simulink model "NGGenset_Test_System"  (Simulink 8.1)
settings: Solver=ode3  SolverMode=SingleTasking  StartTime=0.0  StopTime=150  FixedStep=Ts  RelTol=1e-3
model workspace (MAT data in the model file):
  op_snapshot1 : opcond.OperatingPoint (value not decoded)
PostLoadFcn:
  | Ts=50e-6;SIM_HIL=0;
InitFcn:
  | Ts=50e-6;SIM_HIL=0;
undefined symbols (not defined in the file or in its folder): Gen_900kW_external_control, HIL_GenSet, Left, type, V
libraries: powerlib x31, powerlib_extras x24, simulink x10, dspsigops x6, breakers_1ph_3ph x6, rtio_generic_modbus x6, cables_lib x5, rtlab x2, ssn_lib x2, artemis x1, NG_Genset_lib x1
(part 1 of 3)
settings Model: ARTEMISmethode_block_infos=$$__separator__$$NGGenset_Test_System/ARTEMIS Guide$$__separator__$$  Creator=CH24070  LastModifiedBy=ed12083
settings OptimizationCC: BlockReduction=off  BooleanDataType=off  ExpressionDepthLimit=128
settings DebuggingCC: SaveWithParameterizedLinksMsg=none  SignalResolutionControl=TryResolveAllWithWarning  SolverPrmCheckMsg=none  MultiTaskDSMMsg=warning  MultiTaskCondExecSysMsg=none  FcnCallInpInsideContextMsg=EnableAllAsError  StrictBusMsg=None
settings HardwareCC: TargetUnknown=on
settings RTWCC: IncludeERTFirstTime=on
settings GRTTargetCC: CombineOutputUpdateFcns=on  GRTInterface=off

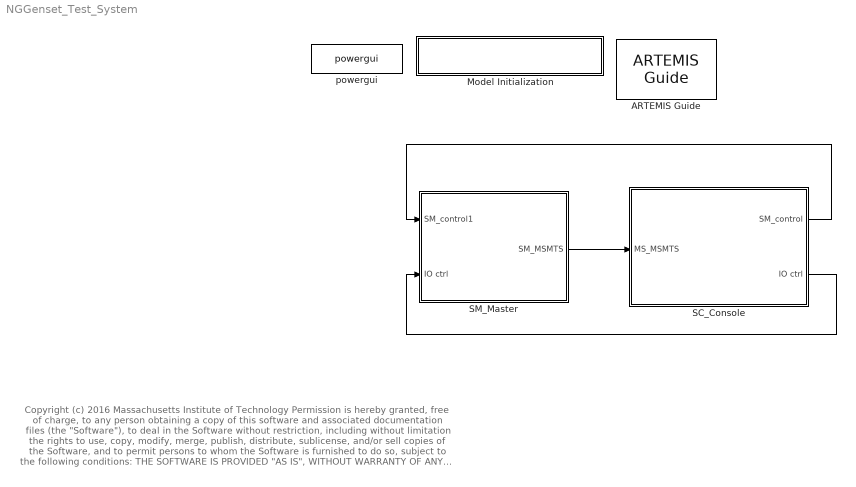
== system NGGenset_Test_System ==
  note: Copyright (c) 2016 Massachusetts Institute of Technology
      | Permission is hereby granted, free of charge, to any person obtaining a copy of this software and associated documentation files (the "Software"), to deal
      | in the Software without restriction, including without limitation the rights to use, copy, modify, merge, publish, distribute, sublicense, and/or sell copies of the
      | Software, and to permit persons to whom the Software is furnished to do so, subject to the following conditions:
      |
      | THE SOFTWARE IS PROVIDED "AS IS", WITHOUT WARRANTY OF ANY KIND, EXPRESS OR IMPLIED, INCLUDING BUT NOT LIMITED TO THE
      | WARRANTIES OF MERCHANTABILITY, FITNESS FOR A PARTICULAR PURPOSE AND NONINFRINGEMENT. IN NO EVENT SHALL THE AUTHORS
      | OR COPYRIGHT HOLDERS BE LIABLE FOR ANY CLAIM, DAMAGES OR OTHER LIABILITY, WHETHER IN AN ACTION OF CONTRACT, TORT OR
      | OTHERWISE, ARISING FROM, OUT OF OR IN CONNECTION WITH THE SOFTWARE OR THE USE OR OTHER DEALINGS IN THE SOFTWARE.
  ARTEMIS Guide : artemis/ARTEMIS/ARTEMIS Guide  Tag=FTSSmethode_opal_4hx0r99  Description=5.0_z1  lock=on  Ts=Ts  opt=art5  dyna=off  nb_perm=4  RT_fullcomp=off  ssn=on  ssn_itvc=off  ssn_ivic=off  ssn_ext=off  ssn_solver=Art5 with Backward Euler nodal interface  ssn_impulse=off  ssn_quasimpulse=off  ssn_impulse_loop=2  paraExtinctionThy=off  Thy_Impulse=on  dtc=Off  dtc_opt=normal  ao=on  simtype=off  ct_mac=off  lin_mov=off  lsp=[0.001 2]  spike_skip=Disabled  dtc_extra=1  dtc_sws=normal  dtc_pied=0.5  SPSRulesBlock=SPSRules  tre=on  ctmm=off  LF=off  dpl_type=ARTEMiS DPL  rlc_type=off  custom_type=off  para=on  ssn_ImpulseLoopBlockedStateUpdate=2  ssn_mov_iter_number=5  ssn_switch_iter_number=5
  Model Initialization : Subsystem  AncestorBlock=artemis/Tools /Misc/Model Initialization  mask(Model Functions){InitFcnX=Ts=50e-6;SIM_HIL=0;, prel=off, posl=on, inif=on, strf=off}
      mask prompts: InitFcnX "Initialisation"; prel "Preload Function"; posl "PostLoad Function"; inif "InitFcn"; strf "StartFcn"
      mask init:
      | currentBlock = gcb;
      | root = bdroot(currentBlock);
      | 
      | if ~strcmp(get_param(root,'BlockDiagramType'),'library')
      |     if prel==1
      |         set_param(root, 'PreLoadFcn', InitFcnX);
      |     else
      |         set_param(root, 'PreLoadFcn', '');
      |     end
      |     if inif==1
      |         set_param(root, 'InitFcn', InitFcnX);
      |     else
      |         set_param(root, 'InitFcn', '');
      |     end
      |     if strf==1
      |         set_param(root, 'StartFcn', InitFcnX);
      |     else
      |         set_param(root, 'StartFcn', '');
      |     end
      |     if posl==1
      |         set_param(root, 'PostLoadFcn', InitFcnX);
      |     else
      |         set_param(root, 'PostLoadFcn', '');
      |     end
      | end
      | 
      | pos = get_param(currentBlock, 'Position');
      | width = pos(3) - pos(1); height = pos(4) - pos(2);
      | txt = [ upper(root) '\n' '- InitFcn. . . . . '  get_param(root, 'InitFcn') ];
      settings: CopyFcn=set_param(gcb,'LinkStatus','inactive')
      mask Display: text(5, height*0.5, txt, 'horizontalAlignment', 'left', 'verticalAlignment', 'middle') ;
  SC_Console : Subsystem
  SM_Master : Subsystem
  powergui : powerlib/powergui  Priority=2  SimulationMode=Discrete  SolverType=Tustin  SampleTime=Ts  frequency=60  SPID=off  DisableSnubberDevices=off  DisableRonSwitches=off  DisableVfSwitches=off  SwTol=0  Interpol=off  DisplayEquations=off  frequencyindice=60  Pbase=100e6  ErrMax=1e-4  Iterations=50  UnitsV=kV  UnitsW=MW  FunctionMessages=off  echomessages=off  HookPort=off  EnableUseOfTLC=off  x0status=blocks  RestoreLinks=warning  ResistiveCurrentMeasurement=off  Frange=logspace(0,3,50)  Ylog=off  Xlog=off  ShowGrid=off  save=off  variable=ZData  structure=0  ZoomFFT=on  StartTime=0.0  cycles=2  DisplayStyle=off  fundamental=60  FreqAxis=off  MaxFrequency=1000  frequencyindicesteady=1  RmsSteady=1  display=off  Ts=0  methode=off
  wires:
  SM_Master/1(SM_MSMTS) -> SC_Console/1(MS_MSMTS)
  SC_Console/1(SM_control) -> SM_Master/1(SM_control1)
  SC_Console/2(IO ctrl) -> SM_Master/2(IO ctrl)

== system NGGenset_Test_System/Model Initialization ==

== system NGGenset_Test_System/SC_Console ==
  note: The 'Overruns' value should remain at 0.
      | The 'Ttotal' value should be equal to the
      | model Fixed-Step size.
  MS_MSMTS : Inport
  Bus Selector : BusSelector  OutputSignals=Grid_PRM,Mains1_PRM,GEN_3_5MVA_PRM,Gen1_meas,Digital In,Load1,Load2,Load3,signal12
  Bus Selector{1..4,7..8} (6 alike) : BusSelector  OutputSignals=Grid_Status,sel_787.Grid_Vabc,sel_787.Iabc,sel_787.Grid_P,sel_787.Grid_Q
  Gen1_3.5MVA : Subsystem  AncestorBlock=HIL_GenSet/Gen_900kW_external_control
  OpComm : rtlab/OpComm  nbport=1  groupe_acq=1  subsys_rate=0  st=0  Synchronization=on  Interpolation=on  Threshold=1.0  Missed_Data=off  Sim_Time=off  Samples=off  dynSigOut=off  from_console=0  warning_done=off  writeOpCommFile=off  Offset=off
  Scope Gen1 : Scope  NumInputPorts=4
      settings: ShowLegends=on  TimeRange=150  YMin=-12500~-1100~-1.5e+06~-1.1e+07  YMax=12500~900~600000~1e+06  Decimation=100
  Scope Grid : Scope  NumInputPorts=5
      settings: TimeRange=60  YMin=0~-20000~-20000~-1000000~-1000000  YMax=1~20000~20000~4000000~4000000  SaveName=ScopeData7  Decimation=100
  Scope Load1 : Scope  NumInputPorts=5
      settings: TimeRange=60  YMin=0~-600~-2000~-1000000~-1000000  YMax=1~600~2000~1000000~1000000  SaveName=ScopeData6  Decimation=100
  Scope Load2 : Scope  NumInputPorts=5
      settings: TimeRange=60  YMin=0~-600~-2000~-1000000~-1000000  YMax=1~600~2000~1000000~1000000  SaveName=ScopeData11  Decimation=100
  Scope Load3 : Scope  NumInputPorts=5
      settings: TimeRange=60  YMin=0~-600~-2000~-1000000~-1000000  YMax=1~600~2000~1000000~1000000  SaveName=ScopeData10  Decimation=100
  Scope Mains1 : Scope  NumInputPorts=5
      settings: TimeRange=60  YMin=0~-20000~-20000~-1000000~-1000000  YMax=1~20000~20000~4000000~4000000  SaveName=ScopeData5  Decimation=100
  Woodward : Subsystem
  SM_control : Outport
  IO ctrl : Outport  Port=2
  wires:
  MS_MSMTS/1 -> OpComm/1
  Gen1_3.5MVA/1(S) -> SM_control/1  "Gen1_3.5MVA"
  OpComm/1 -> Bus Selector/1
  Woodward/1(Out1) -> IO ctrl/1
  Bus Selector1/1 -> Scope Grid/1  "<Grid_Status>"
  Bus Selector1/2 -> Scope Grid/2  "<Grid_Vabc>"
  Bus Selector1/3 -> Scope Grid/3  "<Iabc>"
  Bus Selector1/4 -> Scope Grid/4  "<Grid_P>"
  Bus Selector1/5 -> Scope Grid/5  "<Grid_Q>"
  Bus Selector2/1 -> Scope Mains1/1  "<Grid_Status>"
  Bus Selector2/2 -> Scope Mains1/2  "<Grid_Vabc>"
  Bus Selector2/3 -> Scope Mains1/3  "<Iabc>"
  Bus Selector2/4 -> Scope Mains1/4  "<Grid_P>"
  Bus Selector2/5 -> Scope Mains1/5  "<Grid_Q>"
  Bus Selector/1 -> Bus Selector1/1  "<Grid_PRM>"
  Bus Selector/2 -> Bus Selector2/1  "<Mains1_PRM>"
  Bus Selector3/1 -> Scope Load1/1  "<Grid_Status>"
  Bus Selector3/2 -> Scope Load1/2  "<Grid_Vabc>"
  Bus Selector3/3 -> Scope Load1/3  "<Iabc>"
  Bus Selector3/4 -> Scope Load1/4  "<Grid_P>"
  Bus Selector3/5 -> Scope Load1/5  "<Grid_Q>"
  Bus Selector/6 -> Bus Selector3/1  "<Load1>"
  Bus Selector4/2 -> Scope Gen1/1  "<Grid_Vabc>"
  Bus Selector4/3 -> Scope Gen1/2  "<Iabc>"
  Bus Selector4/4 -> Scope Gen1/3  "<Grid_P>"
  Bus Selector4/5 -> Scope Gen1/4  "<Grid_Q>"
  Bus Selector/3 -> Bus Selector4/1  "<GEN_3_5MVA_PRM>"
  Bus Selector/4 -> Woodward/1(Gen1_Primary)  "<Gen1_meas>"
  Bus Selector/5 -> Woodward/2(DIn_Ch00_31)  "<Digital In>"
  Bus Selector7/1 -> Scope Load3/1  "<Grid_Status>"
  Bus Selector7/2 -> Scope Load3/2  "<Grid_Vabc>"
  Bus Selector7/3 -> Scope Load3/3  "<Iabc>"
  Bus Selector7/4 -> Scope Load3/4  "<Grid_P>"
  Bus Selector7/5 -> Scope Load3/5  "<Grid_Q>"
  Bus Selector8/1 -> Scope Load2/1  "<Grid_Status>"
  Bus Selector8/2 -> Scope Load2/2  "<Grid_Vabc>"
  Bus Selector8/3 -> Scope Load2/3  "<Iabc>"
  Bus Selector8/4 -> Scope Load2/4  "<Grid_P>"
  Bus Selector8/5 -> Scope Load2/5  "<Grid_Q>"
  Bus Selector/8 -> Bus Selector7/1  "<Load3>"
  Bus Selector/7 -> Bus Selector8/1  "<Load2>"

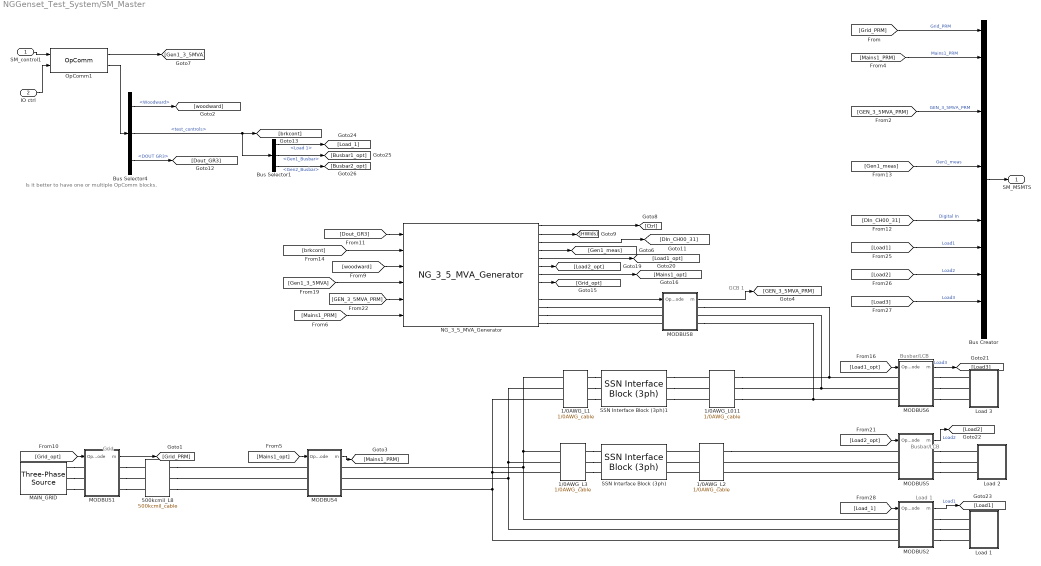
== system NGGenset_Test_System/SM_Master ==
  note: Is it better to have one
      | or multiple OpComm blocks.
  note: GCB 1
  note: Busbar/LCB
  note: Grid
  note: Load 1
  note: Busbar/LCB
  SM_control1 : Inport
  IO ctrl : Inport  Port=2
  1/0AWG_L011 : cables_lib/1//0AWG_cable  length=1000  par_sets=1
  1/0AWG_L1 : cables_lib/1//0AWG_cable  length=1  par_sets=1
  1/0AWG_L2 : cables_lib/1//0AWG_cable  length=1  par_sets=1
  1/0AWG_L3 : cables_lib/1//0AWG_cable  length=1  par_sets=1
  500kcmil_L8 : cables_lib/500kcmil_cable  length=1  par_sets=1
  Bus Creator : BusCreator  Inputs=12
  Bus Selector1 : BusSelector  OutputSignals=Load 1,Gen1_Busbar,Gen2_Busbar
  Bus Selector4 : BusSelector  OutputSignals=Woodward,test_controls,DOUT GR3
  Load 1 : Subsystem  mask{v=13800, kVA=3500*.5, pf=0.90}
      mask prompts: v "VRMSLL"
  Load 2 : Subsystem  mask{v=13800, kVA=3500*.4, pf=0.90}
      mask prompts: v "VRMSLL"
  Load 3 : Subsystem  mask{v=13800, kVA=3500*.1, pf=0.90}
      mask prompts: v "VRMSLL"
  MAIN_GRID : powerlib/Electrical Sources/Three-Phase Source  Voltage=13800  PhaseAngle=0  Frequency=60  InternalConnection=Yg  SpecifyImpedance=on  Resistance=0.8929  Inductance=16.58e-3  ShortCircuitLevel=375e6  BaseVoltage=13800  XRratio=7.9  BusType=swing  Pref=0  Qref=0  Qmin=-inf  Qmax=inf
  MODBUS1 : Subsystem  AncestorBlock=breakers_1ph_3ph/Protection  mask(Protection and Metering){IOC=15E3, TOC=1800, Ts=Ts, VRMSLL=13800, I_nom=200}
      mask prompts: IOC "IOC setting [A]"; TOC "TOC setting [A]"; Ts "Sampling Time [Sec]"; VRMSLL "Nominal Voltage [VRMSLL]"; I_nom "Continous Current [A]"
      mask help:
      | This block simulates the behavior of selected relay functions as well as metering equipment.
      | The block is intended to communicate with a microgrid controller providing it measurements, and switching controls.
      |
      | Supported relay functions (as of 06-15-2015):
      | 50/51: instantaneous and time-inverse overcurrent protection (moderate curve)
      mask Help:
      | This block simulates the behavior of selected relay functions as well as metering equipment (60 Hz - only).
      | The block is intended to communicate with a microgrid controller providing it measurements, and switching controls.
      | 
      | Supported relay functions (as of 06-15-2015):
      | 50/51: instantaneous and time-inverse overcurrent protection (moderate curve)
      | 
      | The input parameters are:
      | 0) Ts:  Sampling time [Seconds]
      | 1) State: 0 for relay logic mode, 1 to close the controlled breaker/switch,
      | and 2 to open the controlled breaker/switch
      | 2) TOC: Time-inverse overcurrent setting [Amperes]
      | 3) IOC: Instantaneous overcurrent setting [Amperes]
      | 
      | Metered parameters are:
      | 0) Status (0-closed, 1-open)
      | 1) Instantaneous voltage (abc)
      | 2) Instantaneous current (abc)
  MODBUS2 : Subsystem  AncestorBlock=breakers_1ph_3ph/Protection  mask(Protection and Metering){IOC=15E3, TOC=1800, Ts=Ts, VRMSLL=13800, I_nom=200}
      mask prompts: IOC "IOC setting [A]"; TOC "TOC setting [A]"; Ts "Sampling Time [Sec]"; VRMSLL "Nominal Voltage [VRMSLL]"; I_nom "Continous Current [A]"
      mask help:
      | This block simulates the behavior of selected relay functions as well as metering equipment.
      | The block is intended to communicate with a microgrid controller providing it measurements, and switching controls.
      |
      | Supported relay functions (as of 06-15-2015):
      | 50/51: instantaneous and time-inverse overcurrent protection (moderate curve)
      mask Help:
      | This block simulates the behavior of selected relay functions as well as metering equipment (60 Hz - only).
      | The block is intended to communicate with a microgrid controller providing it measurements, and switching controls.
      | 
      | Supported relay functions (as of 06-15-2015):
      | 50/51: instantaneous and time-inverse overcurrent protection (moderate curve)
      | 
      | The input parameters are:
      | 0) Ts:  Sampling time [Seconds]
      | 1) State: 0 for relay logic mode, 1 to close the controlled breaker/switch,
      | and 2 to open the controlled breaker/switch
      | 2) TOC: Time-inverse overcurrent setting [Amperes]
      | 3) IOC: Instantaneous overcurrent setting [Amperes]
      | 
      | Metered parameters are:
      | 0) Status (0-closed, 1-open)
      | 1) Instantaneous voltage (abc)
      | 2) Instantaneous current (abc)
  MODBUS4 : Subsystem  AncestorBlock=breakers_1ph_3ph/Protection  mask(Protection and Metering){IOC=15E3, TOC=1800, Ts=Ts, VRMSLL=13800, I_nom=2000}
      mask prompts: IOC "IOC setting [A]"; TOC "TOC setting [A]"; Ts "Sampling Time [Sec]"; VRMSLL "Nominal Voltage [VRMSLL]"; I_nom "Continous Current [A]"
      mask help:
      | This block simulates the behavior of selected relay functions as well as metering equipment.
      | The block is intended to communicate with a microgrid controller providing it measurements, and switching controls.
      |
      | Supported relay functions (as of 06-15-2015):
      | 50/51: instantaneous and time-inverse overcurrent protection (moderate curve)
      mask Help:
      | This block simulates the behavior of selected relay functions as well as metering equipment (60 Hz - only).
      | The block is intended to communicate with a microgrid controller providing it measurements, and switching controls.
      | 
      | Supported relay functions (as of 06-15-2015):
      | 50/51: instantaneous and time-inverse overcurrent protection (moderate curve)
      | 
      | The input parameters are:
      | 0) Ts:  Sampling time [Seconds]
      | 1) State: 0 for relay logic mode, 1 to close the controlled breaker/switch,
      | and 2 to open the controlled breaker/switch
      | 2) TOC: Time-inverse overcurrent setting [Amperes]
      | 3) IOC: Instantaneous overcurrent setting [Amperes]
      | 
      | Metered parameters are:
      | 0) Status (0-closed, 1-open)
      | 1) Instantaneous voltage (abc)
      | 2) Instantaneous current (abc)
  MODBUS5 : Subsystem  AncestorBlock=breakers_1ph_3ph/Protection  mask(Protection and Metering){IOC=15E3, TOC=1800, Ts=Ts, VRMSLL=13800, I_nom=200}
      mask prompts: IOC "IOC setting [A]"; TOC "TOC setting [A]"; Ts "Sampling Time [Sec]"; VRMSLL "Nominal Voltage [VRMSLL]"; I_nom "Continous Current [A]"
      mask help:
      | This block simulates the behavior of selected relay functions as well as metering equipment.
      | The block is intended to communicate with a microgrid controller providing it measurements, and switching controls.
      |
      | Supported relay functions (as of 06-15-2015):
      | 50/51: instantaneous and time-inverse overcurrent protection (moderate curve)
      mask Help:
      | This block simulates the behavior of selected relay functions as well as metering equipment (60 Hz - only).
      | The block is intended to communicate with a microgrid controller providing it measurements, and switching controls.
      | 
      | Supported relay functions (as of 06-15-2015):
      | 50/51: instantaneous and time-inverse overcurrent protection (moderate curve)
      | 
      | The input parameters are:
      | 0) Ts:  Sampling time [Seconds]
      | 1) State: 0 for relay logic mode, 1 to close the controlled breaker/switch,
      | and 2 to open the controlled breaker/switch
      | 2) TOC: Time-inverse overcurrent setting [Amperes]
      | 3) IOC: Instantaneous overcurrent setting [Amperes]
      | 
      | Metered parameters are:
      | 0) Status (0-closed, 1-open)
      | 1) Instantaneous voltage (abc)
      | 2) Instantaneous current (abc)
  MODBUS6 : Subsystem  AncestorBlock=breakers_1ph_3ph/Protection  mask(Protection and Metering){IOC=15E3, TOC=1800, Ts=Ts, VRMSLL=13800, I_nom=200}
      mask prompts: IOC "IOC setting [A]"; TOC "TOC setting [A]"; Ts "Sampling Time [Sec]"; VRMSLL "Nominal Voltage [VRMSLL]"; I_nom "Continous Current [A]"
      mask help:
      | This block simulates the behavior of selected relay functions as well as metering equipment.
      | The block is intended to communicate with a microgrid controller providing it measurements, and switching controls.
      |
      | Supported relay functions (as of 06-15-2015):
      | 50/51: instantaneous and time-inverse overcurrent protection (moderate curve)
      mask Help:
      | This block simulates the behavior of selected relay functions as well as metering equipment (60 Hz - only).
      | The block is intended to communicate with a microgrid controller providing it measurements, and switching controls.
      | 
      | Supported relay functions (as of 06-15-2015):
      | 50/51: instantaneous and time-inverse overcurrent protection (moderate curve)
      | 
      | The input parameters are:
      | 0) Ts:  Sampling time [Seconds]
      | 1) State: 0 for relay logic mode, 1 to close the controlled breaker/switch,
      | and 2 to open the controlled breaker/switch
      | 2) TOC: Time-inverse overcurrent setting [Amperes]
      | 3) IOC: Instantaneous overcurrent setting [Amperes]
      | 
      | Metered parameters are:
      | 0) Status (0-closed, 1-open)
      | 1) Instantaneous voltage (abc)
      | 2) Instantaneous current (abc)
  MODBUS8 : Subsystem  AncestorBlock=breakers_1ph_3ph/Protection  mask(Protection and Metering){IOC=15E3, TOC=1800, Ts=Ts, VRMSLL=13800, I_nom=2000}
      mask prompts: IOC "IOC setting [A]"; TOC "TOC setting [A]"; Ts "Sampling Time [Sec]"; VRMSLL "Nominal Voltage [VRMSLL]"; I_nom "Continous Current [A]"
      mask help:
      | This block simulates the behavior of selected relay functions as well as metering equipment.
      | The block is intended to communicate with a microgrid controller providing it measurements, and switching controls.
      |
      | Supported relay functions (as of 06-15-2015):
      | 50/51: instantaneous and time-inverse overcurrent protection (moderate curve)
      mask Help:
      | This block simulates the behavior of selected relay functions as well as metering equipment (60 Hz - only).
      | The block is intended to communicate with a microgrid controller providing it measurements, and switching controls.
      | 
      | Supported relay functions (as of 06-15-2015):
      | 50/51: instantaneous and time-inverse overcurrent protection (moderate curve)
      | 
      | The input parameters are:
      | 0) Ts:  Sampling time [Seconds]
      | 1) State: 0 for relay logic mode, 1 to close the controlled breaker/switch,
      | and 2 to open the controlled breaker/switch
      | 2) TOC: Time-inverse overcurrent setting [Amperes]
      | 3) IOC: Instantaneous overcurrent setting [Amperes]
      | 
      | Metered parameters are:
      | 0) Status (0-closed, 1-open)
      | 1) Instantaneous voltage (abc)
      | 2) Instantaneous current (abc)
  NG_3_5_MVA_Generator : NG_Genset_lib/NG_3_5_MVA_Generator
  OpComm1 : rtlab/OpComm  nbport=2  groupe_acq=1  subsys_rate=0  st=0  Synchronization=on  Interpolation=on  Threshold=1.0  Missed_Data=off  Sim_Time=off  Samples=off  dynSigOut=off  from_console=1  warning_done=off  writeOpCommFile=off  Offset=off
  SSN Interface Block (3ph) : ssn_lib/SSN Interface Block (3ph)  nb_phase=3  nb_port=2  p1_type=V-type(Left)  p2_type=V-type (Right)  p3_type=V-type(Left)  p4_type=V-type(Left)  p5_type=V-type(Left)  p6_type=V-type(Left)  p7_type=V-type(Left)  p8_type=V-type(Left)  p9_type=V-type(Left)  p10_type=V-type(Left)  p11_type=V-type(Left)  p12_type=V-type(Left)  p13_type=V-type(Left)  p14_type=V-type(Left)  p15_type=V-type(Left)  p16_type=V-type(Left)  I_port_shunt_resistance=1e9
  SSN Interface Block (3ph)1 : ssn_lib/SSN Interface Block (3ph)  nb_phase=3  nb_port=2  p1_type=V-type(Left)  p2_type=V-type (Right)  p3_type=V-type(Left)  p4_type=V-type(Left)  p5_type=V-type(Left)  p6_type=V-type(Left)  p7_type=V-type(Left)  p8_type=V-type(Left)  p9_type=V-type(Left)  p10_type=V-type(Left)  p11_type=V-type(Left)  p12_type=V-type(Left)  p13_type=V-type(Left)  p14_type=V-type(Left)  p15_type=V-type(Left)  p16_type=V-type(Left)  I_port_shunt_resistance=1e9
  SM_MSMTS : Outport
  wires:
  [Grid_PRM] -> Bus Creator/1  "Grid_PRM"
  [GEN_3_5MVA_PRM] -> Bus Creator/4  "GEN_3_5MVA_PRM"
  [Mains1_PRM] -> Bus Creator/2  "Mains1_PRM"
  Bus Creator/1 -> SM_MSMTS/1
  SM_control1/1 -> OpComm1/1
  OpComm1/1 -> [Gen1_3_5MVA]
  OpComm1/2 -> Bus Selector4/1
  Bus Selector4/1 -> [woodward]  "<Woodward>"
  IO ctrl/1 -> OpComm1/2
  Bus Selector4/3 -> [Dout_GR3]  "<DOUT GR3>"
  Bus Selector4/2 -> [brkcont], Bus Selector1/1  "<test_controls>"
  MODBUS1/1(m) -> [Grid_PRM]
  MODBUS8/1(m) -> [GEN_3_5MVA_PRM]
  [Dout_GR3] -> NG_3_5_MVA_Generator/1
  [brkcont] -> NG_3_5_MVA_Generator/2
  NG_3_5_MVA_Generator/4 -> [Gen1_meas]
  NG_3_5_MVA_Generator/1 -> [Ctrl]
  NG_3_5_MVA_Generator/2 -> [HWIds]
  NG_3_5_MVA_Generator/3 -> [DIn_CH00_31]
  [Gen1_3_5MVA] -> NG_3_5_MVA_Generator/4
  [woodward] -> NG_3_5_MVA_Generator/3
  NG_3_5_MVA_Generator/10 -> MODBUS8/1(Op_Mode)
  [Gen1_meas] -> Bus Creator/6  "Gen1_meas"
  [DIn_CH00_31] -> Bus Creator/8  "Digital In"
  NG_3_5_MVA_Generator/8 -> [Grid_opt]
  [Grid_opt] -> MODBUS1/1(Op_Mode)
  NG_3_5_MVA_Generator/7 -> [Mains1_opt]
  [Mains1_PRM] -> NG_3_5_MVA_Generator/6
  NG_3_5_MVA_Generator/6 -> [Load2_opt]
  NG_3_5_MVA_Generator/5 -> [Load1_opt]
  [GEN_3_5MVA_PRM] -> NG_3_5_MVA_Generator/5
  MODBUS4/1(m) -> [Mains1_PRM]
  [Mains1_opt] -> MODBUS4/1(Op_Mode)
  [Load2_opt] -> MODBUS5/1(Op_Mode)
  [Load1_opt] -> MODBUS6/1(Op_Mode)
  MODBUS2/1(m) -> [Load1]  "Load1"
  MODBUS5/1(m) -> [Load2]  "Load2"
  MODBUS6/1(m) -> [Load3]  "Load3"
  [Load1] -> Bus Creator/9  "Load1"
  [Load2] -> Bus Creator/10  "Load2"
  [Load3] -> Bus Creator/11  "Load3"
  Bus Selector1/1 -> [Load_1]  "<Load 1>"
  Bus Selector1/2 -> [Busbar1_opt]  "<Gen1_Busbar>"
  Bus Selector1/3 -> [Busbar2_opt]  "<Gen2_Busbar>"
  [Load_1] -> MODBUS2/1(Op_Mode)
  connections:
  500kcmil_L8/RConn1 -- MODBUS4/LConn1
  500kcmil_L8/RConn2 -- MODBUS4/LConn2
  500kcmil_L8/RConn3 -- MODBUS4/LConn3
  MODBUS8/RConn3 -- MODBUS6/LConn3 -- 1/0AWG_L011/RConn3
  MODBUS1/RConn3 -- 500kcmil_L8/LConn3
  MODBUS1/RConn2 -- 500kcmil_L8/LConn2
  MAIN_GRID/RConn3 -- MODBUS1/LConn3
  MAIN_GRID/RConn2 -- MODBUS1/LConn2
  MAIN_GRID/RConn1 -- MODBUS1/LConn1
  NG_3_5_MVA_Generator/RConn3 -- MODBUS8/LConn3
  NG_3_5_MVA_Generator/RConn2 -- MODBUS8/LConn2
  NG_3_5_MVA_Generator/RConn1 -- MODBUS8/LConn1
  MODBUS2/RConn3 -- Load 1/LConn3
  MODBUS2/RConn2 -- Load 1/LConn2
  MODBUS2/RConn1 -- Load 1/LConn1
  1/0AWG_L1/LConn2 -- MODBUS2/LConn2 -- MODBUS4/RConn2 -- 1/0AWG_L3/LConn2
  MODBUS2/LConn1 -- MODBUS4/RConn1 -- 1/0AWG_L3/LConn1 -- 1/0AWG_L1/LConn1
  1/0AWG_L2/RConn1 -- MODBUS5/LConn1
  MODBUS5/RConn3 -- Load 2/LConn3
  MODBUS5/RConn2 -- Load 2/LConn2
  MODBUS5/RConn1 -- Load 2/LConn1
  MODBUS6/RConn3 -- Load 3/LConn3
  MODBUS6/RConn2 -- Load 3/LConn2
  MODBUS6/RConn1 -- Load 3/LConn1
  SSN Interface Block (3ph)1/RConn1 -- 1/0AWG_L011/LConn1
  SSN Interface Block (3ph)1/RConn2 -- 1/0AWG_L011/LConn2
  SSN Interface Block (3ph)1/RConn3 -- 1/0AWG_L011/LConn3
  1/0AWG_L1/RConn3 -- SSN Interface Block (3ph)1/LConn3
  1/0AWG_L1/RConn2 -- SSN Interface Block (3ph)1/LConn2
  1/0AWG_L1/RConn1 -- SSN Interface Block (3ph)1/LConn1
  MODBUS5/LConn3 -- 1/0AWG_L2/RConn3
  MODBUS5/LConn2 -- 1/0AWG_L2/RConn2
  1/0AWG_L3/RConn3 -- SSN Interface Block (3ph)/LConn3
  1/0AWG_L3/RConn2 -- SSN Interface Block (3ph)/LConn2
  1/0AWG_L3/RConn1 -- SSN Interface Block (3ph)/LConn1
  MODBUS1/RConn1 -- 500kcmil_L8/LConn1
  MODBUS8/RConn1 -- MODBUS6/LConn1 -- 1/0AWG_L011/RConn1
  MODBUS6/LConn2 -- 1/0AWG_L011/RConn2 -- MODBUS8/RConn2
  1/0AWG_L1/LConn3 -- MODBUS2/LConn3 -- MODBUS4/RConn3 -- 1/0AWG_L3/LConn3
  1/0AWG_L2/LConn1 -- SSN Interface Block (3ph)/RConn1
  1/0AWG_L2/LConn2 -- SSN Interface Block (3ph)/RConn2
  1/0AWG_L2/LConn3 -- SSN Interface Block (3ph)/RConn3

== system NGGenset_Test_System/SC_Console/Gen1_3.5MVA ==
  1 - PQ 2 - PV 3 - VF : Constant  Value=3
  2.5 - 130 s : DiscretePulseGenerator  Period=150/Ts  PulseWidth=127.5/Ts  PhaseDelay=2.5/Ts  SampleTime=Ts
  Bus Creator : BusCreator  Inputs=6
  DONOTCHANGE : Constant
  Enable = 1 Disable = 0 : Constant  Value=0
  F : simulink/Math Operations/Slider Gain  low=0.97  gain=1  high=1.03
  Fcmd pu : Constant  Value=1.0
  P : simulink/Math Operations/Slider Gain  low=0  gain=0.8  high=1.1
  Pfactor : Gain  Gain=.9
  Q : simulink/Math Operations/Slider Gain  low=0.01  gain=0.2  high=0.4
  Qfactor : Gain  Gain=.43
  S Profile : simulink/Sources/Repeating Sequence Stair  OutValues=[.1 .1 .1 .1 .1 .1 .1 .1 .1 .1 .1 .1 .1 .1 .5 .5 .5 .5 1 1 1 1 1 ]  tsamp=[5 Ts]  OutMin=[]  OutMax=[]  OutDataTypeStr=Inherit: Inherit via back propagation  OutDataType=fixdt(0,8)  ConRadixGroup=Best Precision: Vector-wise  OutScaling=2^-12
  V : simulink/Math Operations/Slider Gain  low=0.9  gain=1  high=1.1
  VF - to 50s PQ 50 to 110 VF 110 to end : simulink/Sources/Repeating Sequence Stair  OutValues=[3 3 3 3 3 3 3 3 3 3 1 1 1 1 1 1 1 1 1 1 1 1 3 3 3 3 3 3 3 3 3 ]  tsamp=[5 Ts]  OutMin=[]  OutMax=[]  OutDataTypeStr=Inherit: Inherit via back propagation  OutDataType=fixdt(0,8)  ConRadixGroup=Best Precision: Vector-wise  OutScaling=2^-12
  Vcmd pu : Constant
  S : Outport
  wires:
  DONOTCHANGE/1 -> P/1, Q/1, V/1, F/1
  Bus Creator/1 -> S/1
  S Profile/1 -> Qfactor/1, Pfactor/1  "P"
  Qfactor/1 -> Bus Creator/2  "Q"
  Vcmd pu/1 -> Bus Creator/3  "V"
  VF - to 50s PQ 50 to 110 VF 110 to end/1 -> Bus Creator/5  "Mode"
  2.5 - 130 s/1 -> Bus Creator/6  "Enable"
  Fcmd pu/1 -> Bus Creator/4  "F"
  Pfactor/1 -> Bus Creator/1  "P"

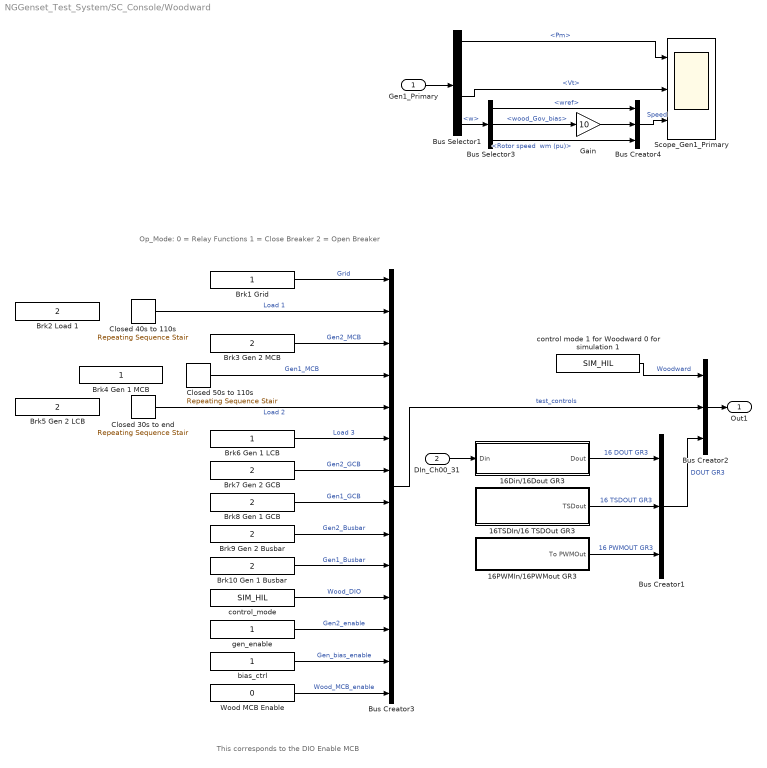
== system NGGenset_Test_System/SC_Console/Woodward ==
  note: Op_Mode:
      | 0 = Relay Functions
      | 1 = Close Breaker
      | 2 = Open Breaker
  note: This corresponds to
      | the DIO Enable MCB
  Gen1_Primary : Inport
  DIn_Ch00_31 : Inport  Port=2
  16Din/16Dout GR3 : Subsystem
  16PWMIn/16PWMout GR3 : Subsystem
  16TSDIn/16 TSDOut GR3 : Subsystem
  Brk1 Grid : Constant
  Brk10 Gen 1 Busbar : Constant  Value=2
  Brk2 Load 1 : Constant  Value=2
  Brk3 Gen 2 MCB : Constant  Value=2
  Brk4 Gen 1 MCB : Constant
  Brk5 Gen 2 LCB : Constant  Value=2
  Brk6 Gen 1 LCB : Constant
  Brk7 Gen 2 GCB : Constant  Value=2
  Brk8 Gen 1 GCB : Constant  Value=2
  Brk9 Gen 2 Busbar : Constant  Value=2
  Bus Creator1 : BusCreator  Inputs=3
  Bus Creator2 : BusCreator  Inputs=3
  Bus Creator3 : BusCreator  Inputs=14
  Bus Creator4 : BusCreator  Inputs=3
  Bus Selector1 : BusSelector  OutputSignals=Pm,Vf,Vt,w
  Bus Selector3 : BusSelector  OutputSignals="wref,w.wood_Gov_bias,w.Rotor speed  wm (pu)"
  Closed 30s to end : simulink/Sources/Repeating Sequence Stair  OutValues=[2 2 2 2 2 2 1 1 1 1 1 1 1 1 1 1 1 1 1 1 1 1 ]  tsamp=[5 Ts]  OutMin=[]  OutMax=[]  OutDataTypeStr=double  OutputDataTypeScalingMode=double  OutDataType=fixdt(0,8)  ConRadixGroup=Best Precision: Vector-wise  OutScaling=2^-12
  Closed 40s to 110s : simulink/Sources/Repeating Sequence Stair  OutValues=[2 2 2 2 2 2 2 2 1 1 1 1 1 1 1 1 1 1 1 1 1 1 2 2 2]  tsamp=[5 Ts]  OutMin=[]  OutMax=[]  OutDataTypeStr=double  OutputDataTypeScalingMode=double  OutDataType=fixdt(0,8)  ConRadixGroup=Best Precision: Vector-wise  OutScaling=2^-12
  Closed 50s to 110s : simulink/Sources/Repeating Sequence Stair  OutValues=[2 2 2 2 2 2 2 2 2 2 1 1 1 1 1 1 1 1 1 1 1 1 2 2 2 2 2]  tsamp=[5 Ts]  OutMin=[]  OutMax=[]  OutDataTypeStr=double  OutputDataTypeScalingMode=double  OutDataType=fixdt(0,8)  ConRadixGroup=Best Precision: Vector-wise  OutScaling=2^-12
  Gain : Gain  Gain=10
  Scope_Gen1_Primary : Scope  NumInputPorts=3
      settings: ShowLegends=on  TimeRange=150  YMin=-0.025~0~0  YMax=0.45~1.05~1.2  SaveName=ScopeData4  Decimation=100
  Wood MCB Enable : Constant  Value=0
  bias_ctrl : Constant
  control mode 1 for Woodward 0 for simulation 1 : Constant  Value=SIM_HIL
  control_mode : Constant  Value=SIM_HIL
  gen_enable : Constant
  Out1 : Outport
  wires:
  control mode 1 for Woodward 0 for simulation 1/1 -> Bus Creator2/1  "Woodward"
  16Din/16Dout GR3/1(Dout) -> Bus Creator1/1  "16 DOUT GR3"
  16TSDIn/16 TSDOut GR3/1(TSDout) -> Bus Creator1/2  "16 TSDOUT GR3"
  16PWMIn/16PWMout GR3/1(To PWMOut) -> Bus Creator1/3  "16 PWMOUT GR3"
  Bus Creator1/1 -> Bus Creator2/3  "DOUT GR3"
  Bus Creator3/1 -> Bus Creator2/2  "test_controls"
  Closed 40s to 110s/1 -> Bus Creator3/2  "Load 1"
  Brk3 Gen 2 MCB/1 -> Bus Creator3/3  "Gen2_MCB"
  Closed 50s to 110s/1 -> Bus Creator3/4  "Gen1_MCB"
  control_mode/1 -> Bus Creator3/11  "Wood_DIO"
  gen_enable/1 -> Bus Creator3/12  "Gen2_enable"
  bias_ctrl/1 -> Bus Creator3/13  "Gen_bias_enable"
  Bus Creator2/1 -> Out1/1
  DIn_Ch00_31/1 -> 16Din/16Dout GR3/1(Din)
  Bus Selector1/1 -> Scope_Gen1_Primary/1  "<Pm>"
  Bus Selector1/3 -> Scope_Gen1_Primary/2  "<Vt>"
  Gen1_Primary/1 -> Bus Selector1/1
  Wood MCB Enable/1 -> Bus Creator3/14  "Wood_MCB_enable"
  Bus Selector1/4 -> Bus Selector3/1  "<w>"
  Bus Selector3/1 -> Bus Creator4/1  "<wref>"
  Bus Selector3/2 -> Gain/1  "<wood_Gov_bias>"
  Bus Selector3/3 -> Bus Creator4/3  "<Rotor speed  wm (pu)>"
  Closed 30s to end/1 -> Bus Creator3/5  "Load 2"
  Brk6 Gen 1 LCB/1 -> Bus Creator3/6  "Load 3"
  Brk7 Gen 2 GCB/1 -> Bus Creator3/7  "Gen2_GCB"
  Brk8 Gen 1 GCB/1 -> Bus Creator3/8  "Gen1_GCB"
  Gain/1 -> Bus Creator4/2
  Brk9 Gen 2 Busbar/1 -> Bus Creator3/9  "Gen2_Busbar"
  Brk10 Gen 1 Busbar/1 -> Bus Creator3/10  "Gen1_Busbar"
  Brk1 Grid/1 -> Bus Creator3/1  "Grid"
  Bus Creator4/1 -> Scope_Gen1_Primary/3  "Speed"

== system NGGenset_Test_System/SM_Master/Load 1 ==
  Constant Load : powerlib/Elements/Three-Phase Parallel RLC Load  LConnTagsString=A|B|C  Configuration=Y (grounded)  NominalVoltage=v  NominalFrequency=60  ActivePower=kVA*1E3*pf  InductivePower=kVA*1E3*sqrt(1-pf^2)  CapacitivePower=0  Measurements=None  LoadType=constant Z
  A : PMIOPort  Port=1  Side=Left
  B : PMIOPort  Port=2  Side=Left
  C : PMIOPort  Port=3  Side=Left
  connections:
  Constant Load/LConn1 -- A/RConn1
  B/RConn1 -- Constant Load/LConn2
  C/RConn1 -- Constant Load/LConn3

== system NGGenset_Test_System/SM_Master/Load 2 ==
  Constant Load : powerlib/Elements/Three-Phase Parallel RLC Load  LConnTagsString=A|B|C  Configuration=Y (grounded)  NominalVoltage=v  NominalFrequency=60  ActivePower=kVA*1E3*pf  InductivePower=kVA*1E3*sqrt(1-pf^2)  CapacitivePower=0  Measurements=None  LoadType=constant Z
  A : PMIOPort  Port=1  Side=Left
  B : PMIOPort  Port=2  Side=Left
  C : PMIOPort  Port=3  Side=Left
  connections:
  Constant Load/LConn1 -- A/RConn1
  B/RConn1 -- Constant Load/LConn2
  C/RConn1 -- Constant Load/LConn3

== system NGGenset_Test_System/SM_Master/Load 3 ==
  Constant Load : powerlib/Elements/Three-Phase Parallel RLC Load  LConnTagsString=A|B|C  Configuration=Y (grounded)  NominalVoltage=v  NominalFrequency=60  ActivePower=kVA*1E3*pf  InductivePower=kVA*1E3*sqrt(1-pf^2)  CapacitivePower=0  Measurements=None  LoadType=constant Z
  A : PMIOPort  Port=1  Side=Left
  B : PMIOPort  Port=2  Side=Left
  C : PMIOPort  Port=3  Side=Left
  connections:
  Constant Load/LConn1 -- A/RConn1
  B/RConn1 -- Constant Load/LConn2
  C/RConn1 -- Constant Load/LConn3

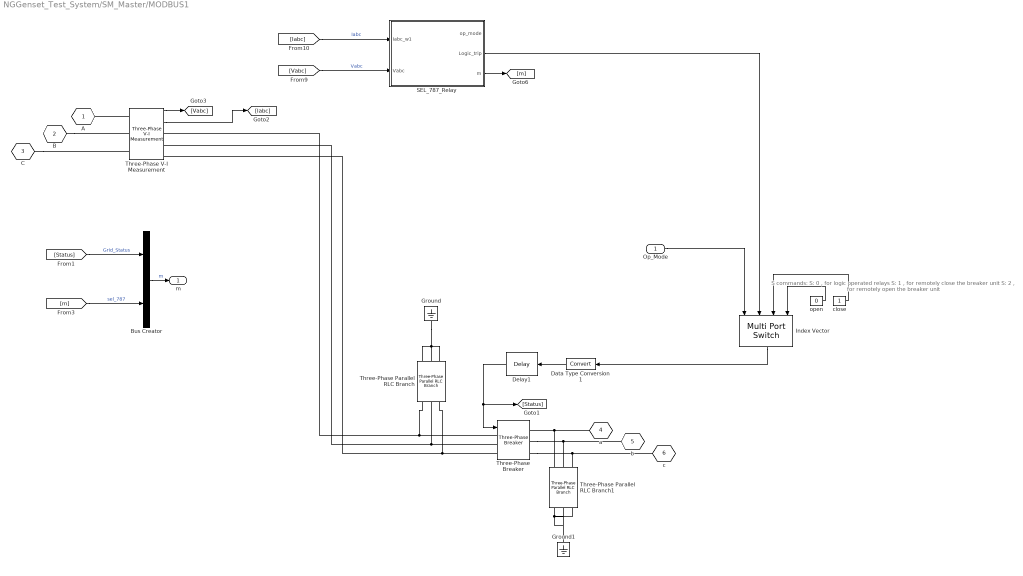
== system NGGenset_Test_System/SM_Master/MODBUS1 ==
  note: S commands:
      | S: 0 , for logic operated relays
      | S: 1 ,  for remotely close the breaker unit
      | S: 2 , for remotely open the breaker unit
  Op_Mode : Inport
  Bus Creator : BusCreator  Inputs=2
  Data Type Conversion1 : DataTypeConversion
  Delay1 : dspsigops/Delay  dly_unit=Samples  delay=lower((3/60)/Ts)  ic_detail=off  dif_ic_for_ch=off  dif_ic_for_dly=off  ic=1  reset_popup=None
  Ground : powerlib/Elements/Ground  LConnTagsString=a
  Ground1 : powerlib/Elements/Ground  LConnTagsString=a
  Index Vector : MultiPortSwitch  DataPortOrder=Zero-based contiguous  DataPortIndices={2,1,0}  zeroidx=on
  SEL_787_Relay : Subsystem
  Three-Phase Parallel RLC Branch : powerlib/Elements/Three-Phase Parallel RLC Branch  LConnTagsString=A|B|C  RConnTagsString=A|B|C  BranchType=R  Resistance=10e6  Inductance=1e-3  Capacitance=1e-6  Measurements=None
  Three-Phase Parallel RLC Branch1 : powerlib/Elements/Three-Phase Parallel RLC Branch  LConnTagsString=A|B|C  RConnTagsString=A|B|C  BranchType=R  Resistance=10e6  Inductance=1e-3  Capacitance=1e-6  Measurements=None
  Three-Phase V-I Measurement : powerlib/Measurements/Three-Phase V-I Measurement  VoltageMeasurement=phase-to-ground  SetLabelV=off  LabelV=Vabc  Vpu=off  VpuLL=off  CurrentMeasurement=yes  SetLabelI=off  LabelI=Iabc  Ipu=off  Pbase=100e6  Vbase=500e3  OutputType=Complex  PhasorSimulation=off  PSBequivalent=0
  Three-Phase Breaker : powerlib/Elements/Three-Phase Breaker  InitialState=closed  SwitchA=on  SwitchB=on  SwitchC=on  SwitchTimes="[1/60  5/60]"  External=on  BreakerResistance=1e-3  SnubberResistance=0  SnubberCapacitance=0  Measurements=None
  close : Constant
  open : Constant  Value=0
  A : PMIOPort  Tag=PMCPort  Port=1  Side=Left
  B : PMIOPort  Tag=PMCPort  Port=2  Side=Left
  C : PMIOPort  Tag=PMCPort  Port=3  Side=Left
  a : PMIOPort  Tag=PMCPort  Port=4  Side=Right
  b : PMIOPort  Tag=PMCPort  Port=5  Side=Right
  c : PMIOPort  Tag=PMCPort  Port=6  Side=Right
  m : Outport
  wires:
  [m] -> Bus Creator/2  "sel_787"
  SEL_787_Relay/3(m) -> [m]
  Bus Creator/1 -> m/1  "m"
  [Status] -> Bus Creator/1  "Grid_Status"
  Delay1/1 -> [Status], Three-Phase Breaker/1
  Three-Phase V-I Measurement/1 -> [Vabc]
  Three-Phase V-I Measurement/2 -> [Iabc]
  open/1 -> Index Vector/4
  close/1 -> Index Vector/3
  Index Vector/1 -> Data Type Conversion1/1
  Data Type Conversion1/1 -> Delay1/1
  [Iabc] -> SEL_787_Relay/1(Iabc_w1)  "Iabc"
  [Vabc] -> SEL_787_Relay/2(Vabc)  "Vabc"
  SEL_787_Relay/2(Logic_trip) -> Index Vector/2
  Op_Mode/1 -> Index Vector/1
  connections:
  Three-Phase Breaker/LConn1 -- Three-Phase V-I Measurement/RConn1 -- Three-Phase Parallel RLC Branch/RConn1
  Three-Phase Breaker/LConn2 -- Three-Phase V-I Measurement/RConn2 -- Three-Phase Parallel RLC Branch/RConn2
  Three-Phase Breaker/LConn3 -- Three-Phase V-I Measurement/RConn3 -- Three-Phase Parallel RLC Branch/RConn3
  Three-Phase Breaker/RConn2 -- b/RConn1 -- Three-Phase Parallel RLC Branch1/RConn2
  Three-Phase Breaker/RConn3 -- c/RConn1 -- Three-Phase Parallel RLC Branch1/RConn3
  Three-Phase V-I Measurement/LConn1 -- A/RConn1
  a/RConn1 -- Three-Phase Breaker/RConn1 -- Three-Phase Parallel RLC Branch1/RConn1
  C/RConn1 -- Three-Phase V-I Measurement/LConn3
  B/RConn1 -- Three-Phase V-I Measurement/LConn2
  Three-Phase Parallel RLC Branch1/LConn1 -- Ground1/LConn1 -- Three-Phase Parallel RLC Branch1/LConn2 -- Three-Phase Parallel RLC Branch1/LConn3
  Ground/LConn1 -- Three-Phase Parallel RLC Branch/LConn2 -- Three-Phase Parallel RLC Branch/LConn3 -- Three-Phase Parallel RLC Branch/LConn1

== system NGGenset_Test_System/SM_Master/MODBUS2 ==
  note: S commands:
      | S: 0 , for logic operated relays
      | S: 1 ,  for remotely close the breaker unit
      | S: 2 , for remotely open the breaker unit
  Op_Mode : Inport
  Bus Creator : BusCreator  Inputs=2
  Data Type Conversion1 : DataTypeConversion
  Delay1 : dspsigops/Delay  dly_unit=Samples  delay=lower((3/60)/Ts)  ic_detail=off  dif_ic_for_ch=off  dif_ic_for_dly=off  ic=1  reset_popup=None
  Ground : powerlib/Elements/Ground  LConnTagsString=a
  Index Vector : MultiPortSwitch  DataPortOrder=Zero-based contiguous  DataPortIndices={2,1,0}  zeroidx=on
  SEL_787_Relay : Subsystem
  Three-Phase Parallel RLC Branch : powerlib/Elements/Three-Phase Parallel RLC Branch  LConnTagsString=A|B|C  RConnTagsString=A|B|C  BranchType=R  Resistance=10e6  Inductance=1e-3  Capacitance=1e-6  Measurements=None
  Three-Phase V-I Measurement : powerlib/Measurements/Three-Phase V-I Measurement  VoltageMeasurement=phase-to-ground  SetLabelV=off  LabelV=Vabc  Vpu=off  VpuLL=off  CurrentMeasurement=yes  SetLabelI=off  LabelI=Iabc  Ipu=off  Pbase=100e6  Vbase=500e3  OutputType=Complex  PhasorSimulation=off  PSBequivalent=0
  Three-Phase Breaker : powerlib/Elements/Three-Phase Breaker  InitialState=open  SwitchA=on  SwitchB=on  SwitchC=on  SwitchTimes="[1/60  5/60]"  External=on  BreakerResistance=1e-3  SnubberResistance=0  SnubberCapacitance=0  Measurements=None
  close : Constant
  open : Constant  Value=0
  A : PMIOPort  Tag=PMCPort  Port=1  Side=Left
  B : PMIOPort  Tag=PMCPort  Port=2  Side=Left
  C : PMIOPort  Tag=PMCPort  Port=3  Side=Left
  a : PMIOPort  Tag=PMCPort  Port=4  Side=Right
  b : PMIOPort  Tag=PMCPort  Port=5  Side=Right
  c : PMIOPort  Tag=PMCPort  Port=6  Side=Right
  m : Outport
  wires:
  [m] -> Bus Creator/2  "sel_787"
  SEL_787_Relay/3(m) -> [m]
  Bus Creator/1 -> m/1  "m"
  [Status] -> Bus Creator/1  "Grid_Status"
  Delay1/1 -> [Status], Three-Phase Breaker/1
  Three-Phase V-I Measurement/1 -> [Vabc]
  Three-Phase V-I Measurement/2 -> [Iabc]
  open/1 -> Index Vector/4
  close/1 -> Index Vector/3
  Index Vector/1 -> Data Type Conversion1/1
  Data Type Conversion1/1 -> Delay1/1
  [Iabc] -> SEL_787_Relay/1(Iabc_w1)  "Iabc"
  [Vabc] -> SEL_787_Relay/2(Vabc)  "Vabc"
  SEL_787_Relay/2(Logic_trip) -> Index Vector/2
  Op_Mode/1 -> Index Vector/1
  connections:
  Three-Phase V-I Measurement/RConn1 -- Three-Phase Parallel RLC Branch/RConn1 -- Three-Phase Breaker/LConn1
  Three-Phase V-I Measurement/RConn2 -- Three-Phase Parallel RLC Branch/RConn2 -- Three-Phase Breaker/LConn2
  Three-Phase V-I Measurement/RConn3 -- Three-Phase Parallel RLC Branch/RConn3 -- Three-Phase Breaker/LConn3
  Three-Phase Breaker/RConn2 -- b/RConn1
  Three-Phase Breaker/RConn3 -- c/RConn1
  Three-Phase V-I Measurement/LConn1 -- A/RConn1
  a/RConn1 -- Three-Phase Breaker/RConn1
  C/RConn1 -- Three-Phase V-I Measurement/LConn3
  B/RConn1 -- Three-Phase V-I Measurement/LConn2
  Ground/LConn1 -- Three-Phase Parallel RLC Branch/LConn2 -- Three-Phase Parallel RLC Branch/LConn3 -- Three-Phase Parallel RLC Branch/LConn1

== system NGGenset_Test_System/SM_Master/MODBUS4 ==
  note: S commands:
      | S: 0 , for logic operated relays
      | S: 1 ,  for remotely close the breaker unit
      | S: 2 , for remotely open the breaker unit
  Op_Mode : Inport
  Bus Creator : BusCreator  Inputs=2
  Data Type Conversion1 : DataTypeConversion
  Delay1 : dspsigops/Delay  dly_unit=Samples  delay=lower((3/60)/Ts)  ic_detail=off  dif_ic_for_ch=off  dif_ic_for_dly=off  ic=1  reset_popup=None
  Ground : powerlib/Elements/Ground  LConnTagsString=a
  Index Vector : MultiPortSwitch  DataPortOrder=Zero-based contiguous  DataPortIndices={2,1,0}  zeroidx=on
  SEL_787_Relay : Subsystem
  Three-Phase Parallel RLC Branch : powerlib/Elements/Three-Phase Parallel RLC Branch  LConnTagsString=A|B|C  RConnTagsString=A|B|C  BranchType=R  Resistance=10e6  Inductance=1e-3  Capacitance=1e-6  Measurements=None
  Three-Phase V-I Measurement : powerlib/Measurements/Three-Phase V-I Measurement  VoltageMeasurement=phase-to-ground  SetLabelV=off  LabelV=Vabc  Vpu=off  VpuLL=off  CurrentMeasurement=yes  SetLabelI=off  LabelI=Iabc  Ipu=off  Pbase=100e6  Vbase=500e3  OutputType=Complex  PhasorSimulation=off  PSBequivalent=0
  Three-Phase Breaker : powerlib/Elements/Three-Phase Breaker  InitialState=open  SwitchA=on  SwitchB=on  SwitchC=on  SwitchTimes="[1/60  5/60]"  External=on  BreakerResistance=1e-3  SnubberResistance=0  SnubberCapacitance=0  Measurements=None
  close : Constant
  open : Constant  Value=0
  A : PMIOPort  Tag=PMCPort  Port=1  Side=Left
  B : PMIOPort  Tag=PMCPort  Port=2  Side=Left
  C : PMIOPort  Tag=PMCPort  Port=3  Side=Left
  a : PMIOPort  Tag=PMCPort  Port=4  Side=Right
  b : PMIOPort  Tag=PMCPort  Port=5  Side=Right
  c : PMIOPort  Tag=PMCPort  Port=6  Side=Right
  m : Outport
  wires:
  [m] -> Bus Creator/2  "sel_787"
  SEL_787_Relay/3(m) -> [m]
  Bus Creator/1 -> m/1  "m"
  [Status] -> Bus Creator/1  "Grid_Status"
  Delay1/1 -> [Status], Three-Phase Breaker/1
  Three-Phase V-I Measurement/1 -> [Vabc]
  Three-Phase V-I Measurement/2 -> [Iabc]
  open/1 -> Index Vector/4
  close/1 -> Index Vector/3
  Index Vector/1 -> Data Type Conversion1/1
  Data Type Conversion1/1 -> Delay1/1
  [Iabc] -> SEL_787_Relay/1(Iabc_w1)  "Iabc"
  [Vabc] -> SEL_787_Relay/2(Vabc)  "Vabc"
  SEL_787_Relay/2(Logic_trip) -> Index Vector/2
  Op_Mode/1 -> Index Vector/1
  connections:
  Three-Phase V-I Measurement/RConn1 -- Three-Phase Parallel RLC Branch/RConn1 -- Three-Phase Breaker/LConn1
  Three-Phase V-I Measurement/RConn2 -- Three-Phase Parallel RLC Branch/RConn2 -- Three-Phase Breaker/LConn2
  Three-Phase V-I Measurement/RConn3 -- Three-Phase Parallel RLC Branch/RConn3 -- Three-Phase Breaker/LConn3
  Three-Phase Breaker/RConn2 -- b/RConn1
  Three-Phase Breaker/RConn3 -- c/RConn1
  Three-Phase V-I Measurement/LConn1 -- A/RConn1
  a/RConn1 -- Three-Phase Breaker/RConn1
  C/RConn1 -- Three-Phase V-I Measurement/LConn3
  B/RConn1 -- Three-Phase V-I Measurement/LConn2
  Ground/LConn1 -- Three-Phase Parallel RLC Branch/LConn2 -- Three-Phase Parallel RLC Branch/LConn3 -- Three-Phase Parallel RLC Branch/LConn1

== system NGGenset_Test_System/SM_Master/MODBUS5 ==
  note: S commands:
      | S: 0 , for logic operated relays
      | S: 1 ,  for remotely close the breaker unit
      | S: 2 , for remotely open the breaker unit
  Op_Mode : Inport
  Bus Creator : BusCreator  Inputs=2
  Data Type Conversion1 : DataTypeConversion
  Delay1 : dspsigops/Delay  dly_unit=Samples  delay=lower((3/60)/Ts)  ic_detail=off  dif_ic_for_ch=off  dif_ic_for_dly=off  ic=1  reset_popup=None
  Ground : powerlib/Elements/Ground  LConnTagsString=a
  Index Vector : MultiPortSwitch  DataPortOrder=Zero-based contiguous  DataPortIndices={2,1,0}  zeroidx=on
  SEL_787_Relay : Subsystem
  Three-Phase Parallel RLC Branch : powerlib/Elements/Three-Phase Parallel RLC Branch  LConnTagsString=A|B|C  RConnTagsString=A|B|C  BranchType=R  Resistance=10e6  Inductance=1e-3  Capacitance=1e-6  Measurements=None
  Three-Phase V-I Measurement : powerlib/Measurements/Three-Phase V-I Measurement  VoltageMeasurement=phase-to-ground  SetLabelV=off  LabelV=Vabc  Vpu=off  VpuLL=off  CurrentMeasurement=yes  SetLabelI=off  LabelI=Iabc  Ipu=off  Pbase=100e6  Vbase=500e3  OutputType=Complex  PhasorSimulation=off  PSBequivalent=0
  Three-Phase Breaker : powerlib/Elements/Three-Phase Breaker  InitialState=open  SwitchA=on  SwitchB=on  SwitchC=on  SwitchTimes="[1/60  5/60]"  External=on  BreakerResistance=1e-3  SnubberResistance=0  SnubberCapacitance=0  Measurements=None
  close : Constant
  open : Constant  Value=0
  A : PMIOPort  Tag=PMCPort  Port=1  Side=Left
  B : PMIOPort  Tag=PMCPort  Port=2  Side=Left
  C : PMIOPort  Tag=PMCPort  Port=3  Side=Left
  a : PMIOPort  Tag=PMCPort  Port=4  Side=Right
  b : PMIOPort  Tag=PMCPort  Port=5  Side=Right
  c : PMIOPort  Tag=PMCPort  Port=6  Side=Right
  m : Outport
  wires:
  [m] -> Bus Creator/2  "sel_787"
  SEL_787_Relay/3(m) -> [m]
  Bus Creator/1 -> m/1  "m"
  [Status] -> Bus Creator/1  "Grid_Status"
  Delay1/1 -> [Status], Three-Phase Breaker/1
  Three-Phase V-I Measurement/1 -> [Vabc]
  Three-Phase V-I Measurement/2 -> [Iabc]
  open/1 -> Index Vector/4
  close/1 -> Index Vector/3
  Index Vector/1 -> Data Type Conversion1/1
  Data Type Conversion1/1 -> Delay1/1
  [Iabc] -> SEL_787_Relay/1(Iabc_w1)  "Iabc"
  [Vabc] -> SEL_787_Relay/2(Vabc)  "Vabc"
  SEL_787_Relay/2(Logic_trip) -> Index Vector/2
  Op_Mode/1 -> Index Vector/1
  connections:
  Three-Phase V-I Measurement/RConn1 -- Three-Phase Parallel RLC Branch/RConn1 -- Three-Phase Breaker/LConn1
  Three-Phase V-I Measurement/RConn2 -- Three-Phase Parallel RLC Branch/RConn2 -- Three-Phase Breaker/LConn2
  Three-Phase V-I Measurement/RConn3 -- Three-Phase Parallel RLC Branch/RConn3 -- Three-Phase Breaker/LConn3
  Three-Phase Breaker/RConn2 -- b/RConn1
  Three-Phase Breaker/RConn3 -- c/RConn1
  Three-Phase V-I Measurement/LConn1 -- A/RConn1
  a/RConn1 -- Three-Phase Breaker/RConn1
  C/RConn1 -- Three-Phase V-I Measurement/LConn3
  B/RConn1 -- Three-Phase V-I Measurement/LConn2
  Ground/LConn1 -- Three-Phase Parallel RLC Branch/LConn2 -- Three-Phase Parallel RLC Branch/LConn3 -- Three-Phase Parallel RLC Branch/LConn1

== system NGGenset_Test_System/SM_Master/MODBUS6 ==
  note: S commands:
      | S: 0 , for logic operated relays
      | S: 1 ,  for remotely close the breaker unit
      | S: 2 , for remotely open the breaker unit
  Op_Mode : Inport
  Bus Creator : BusCreator  Inputs=2
  Data Type Conversion1 : DataTypeConversion
  Delay1 : dspsigops/Delay  dly_unit=Samples  delay=lower((3/60)/Ts)  ic_detail=off  dif_ic_for_ch=off  dif_ic_for_dly=off  ic=1  reset_popup=None
  Ground : powerlib/Elements/Ground  LConnTagsString=a
  Index Vector : MultiPortSwitch  DataPortOrder=Zero-based contiguous  DataPortIndices={2,1,0}  zeroidx=on
  SEL_787_Relay : Subsystem
  Three-Phase Parallel RLC Branch : powerlib/Elements/Three-Phase Parallel RLC Branch  LConnTagsString=A|B|C  RConnTagsString=A|B|C  BranchType=R  Resistance=10e6  Inductance=1e-3  Capacitance=1e-6  Measurements=None
  Three-Phase V-I Measurement : powerlib/Measurements/Three-Phase V-I Measurement  VoltageMeasurement=phase-to-ground  SetLabelV=off  LabelV=Vabc  Vpu=off  VpuLL=off  CurrentMeasurement=yes  SetLabelI=off  LabelI=Iabc  Ipu=off  Pbase=100e6  Vbase=500e3  OutputType=Complex  PhasorSimulation=off  PSBequivalent=0
  Three-Phase Breaker : powerlib/Elements/Three-Phase Breaker  InitialState=open  SwitchA=on  SwitchB=on  SwitchC=on  SwitchTimes="[1/60  5/60]"  External=on  BreakerResistance=1e-3  SnubberResistance=0  SnubberCapacitance=0  Measurements=None
  close : Constant
  open : Constant  Value=0
  A : PMIOPort  Tag=PMCPort  Port=1  Side=Left
  B : PMIOPort  Tag=PMCPort  Port=2  Side=Left
  C : PMIOPort  Tag=PMCPort  Port=3  Side=Left
  a : PMIOPort  Tag=PMCPort  Port=4  Side=Right
  b : PMIOPort  Tag=PMCPort  Port=5  Side=Right
  c : PMIOPort  Tag=PMCPort  Port=6  Side=Right
  m : Outport
  wires:
  [m] -> Bus Creator/2  "sel_787"
  SEL_787_Relay/3(m) -> [m]
  Bus Creator/1 -> m/1  "m"
  [Status] -> Bus Creator/1  "Grid_Status"
  Delay1/1 -> [Status], Three-Phase Breaker/1
  Three-Phase V-I Measurement/1 -> [Vabc]
  Three-Phase V-I Measurement/2 -> [Iabc]
  open/1 -> Index Vector/4
  close/1 -> Index Vector/3
  Index Vector/1 -> Data Type Conversion1/1
  Data Type Conversion1/1 -> Delay1/1
  [Iabc] -> SEL_787_Relay/1(Iabc_w1)  "Iabc"
  [Vabc] -> SEL_787_Relay/2(Vabc)  "Vabc"
  SEL_787_Relay/2(Logic_trip) -> Index Vector/2
  Op_Mode/1 -> Index Vector/1
  connections:
  Three-Phase V-I Measurement/RConn1 -- Three-Phase Parallel RLC Branch/RConn1 -- Three-Phase Breaker/LConn1
  Three-Phase V-I Measurement/RConn2 -- Three-Phase Parallel RLC Branch/RConn2 -- Three-Phase Breaker/LConn2
  Three-Phase V-I Measurement/RConn3 -- Three-Phase Parallel RLC Branch/RConn3 -- Three-Phase Breaker/LConn3
  Three-Phase Breaker/RConn2 -- b/RConn1
  Three-Phase Breaker/RConn3 -- c/RConn1
  Three-Phase V-I Measurement/LConn1 -- A/RConn1
  a/RConn1 -- Three-Phase Breaker/RConn1
  C/RConn1 -- Three-Phase V-I Measurement/LConn3
  B/RConn1 -- Three-Phase V-I Measurement/LConn2
  Ground/LConn1 -- Three-Phase Parallel RLC Branch/LConn2 -- Three-Phase Parallel RLC Branch/LConn3 -- Three-Phase Parallel RLC Branch/LConn1
